simulink model "cartpole"  (R2019b)
settings: Solver=ode15s  StartTime=0.0  StopTime=10  MaxStep=0.01  RelTol=1e-3  EnableMultiTasking=on
values from neighbouring files (symbols this model uses):
  cartpole_init_pose = [-(ground.w/2-1) tire.r+ground.l/2 0]    [cartpole_conf.m]
  g = 9.81    [cartpole_conf.m]
  m_cart = body.m + 2*tire.m + 4*omni.m    [cartpole_conf.m]
  max_steer = 0.42    [cartpole_conf.m]
  max_v = 1    [cartpole_conf.m]
  path = [4.0 0.0 2.0]    [cartpole_conf.m]
  tread = tire.l + body.h    [cartpole_conf.m]
  waypoint_length = 0.05    [cartpole_conf.m]
undefined symbols (not defined in the file or in its folder): body, Body, ground, Ground, LBomni, LCtire, LFomni, omni, RBomni, RCtire, RFomni, sigbuilder_block, stick, Stick, tire, Wall1, Wall2, Wall3, Wall4, X, Y, Z
libraries: sm_lib x106, nesl_utility x18, simulink x5
(part 1 of 4)
settings Model: NumberOfSteps=10  EnablePacing=on  PacingRate=1000  Creator=土屋　一朗  LastModifiedBy=wataru
settings DataIOCC: LimitDataPoints=on  MaxDataPoints=10000
settings OptimizationCC: LifeSpan=inf
settings DebuggingCC: AllowSymbolicDim=off  SFUnexpectedBacktrackingDiag=warning  SFNoUnconditionalDefaultTransitionDiag=warning  SFExecutionAtInitializationDiag=none  ArithmeticOperatorsInVariantConditions=warning
settings SFSimCC: SimUseLocalCustomCode=off  CustomCodeUndefinedFunction=UseInterfaceOnly
settings RTWCC: RTWUseLocalCustomCode=off
settings CodeAppCC: StateflowObjectComments=on
settings GRTTargetCC: TargetLangStandard=C89/C90 (ANSI)  GeneratePreprocessorConditionals=Disable all
settings ConfigComp: CovMetricSettings=dw  CovHtmlReporting=on  CovSaveCumulativeToWorkspaceVar=on  CovSaveSingleToWorkspaceVar=on  CovExternalEMLEnable=off  CovSFcnEnable=off
settings SimscapeCC: SimscapeLogType=all  SimscapeLogSimulationStatistics=on  SimscapeLogDataHistory=10000
settings ExplorerConfigSet: InternalSimMechanicsExplorerSettings="<ExplorerConfiguration><canonicalview>planar_xy</canonicalview><AnimationSetting><BasePlaybackSpeed>1.0</BasePlaybackSpeed><PlaybackSpeedFactor>1.0</PlaybackSpeedFactor></AnimationSetting><TilePanel><TileInfo><Tiles Columns=\"1\" Count=\"1\" Rows=\"1\"><Column Weight=\"1\"/><Row Weight=\"1\"/><Tile Height=\"1\" Width=\"1\" X=\"0\" Y=\"0\"/></Tiles></TileInfo><SceneInfo><SceneViewer><BGColor><R>0.60000002384185791</R><G>0.60000002384185791</G><B>0.60000002384185791</B></BGColor><Camera><DoPerspective>off</DoPerspective><Position><X>5.81087438691202873</X><Y>6.21087454411730366</Y><Z>5.81087458520799416</Z></Position><Center><X>1.96953159822821355e-07</X><Y>0.400000354158434546</Y><Z>3.9524912481825325e-07</Z></Center><Up><X>-0.408248290463863073</X><Y>0.816496580927726145</Y><Z>-0.408248290463863073</Z></Up><ViewLimDist>1</ViewLimDist><YLim>7.91620397355392402</YLim><XLim>7.39244756698608452</XLim></Camera></SceneViewer></SceneInfo></TilePanel><MechEditorPanel><Cameras/><GfxPanelCameraMap/><VideoCreator><PlaybackSpeedRatio>1.0</PlaybackSpeedRatio><FrameRate>30</FrameRate><VideoFormat>Motion JPEG AVI</VideoFormat><FrameSize>auto</FrameSize></VideoCreator></MechEditorPanel></ExplorerConfiguration>"

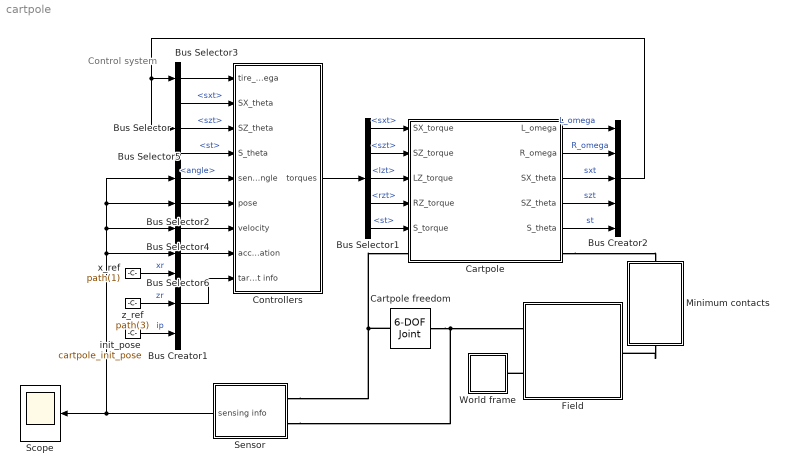
== system cartpole ==
  note: Control system
  Bus Creator1 : BusCreator  Inputs=3
  Bus Creator2 : BusCreator  Inputs=5
  Bus Selector : BusSelector  OutputSignals=sxt,szt,st
  Bus Selector1 : BusSelector  OutputSignals=sxt,szt,lzt,rzt,st
  Bus Selector2 : BusSelector  OutputSignals=x,z  OutputAsBus=on
  Bus Selector3 : BusSelector  OutputSignals=L_omega,R_omega  OutputAsBus=on
  Bus Selector4 : BusSelector  OutputSignals=vx,vz  OutputAsBus=on
  Bus Selector5 : BusSelector  OutputSignals=angle
  Bus Selector6 : BusSelector  OutputSignals=ax,az  OutputAsBus=on
  Cartpole : Subsystem  mask{s_m=stick.m, s_w=stick.w, s_l=stick.l, s_h=stick.h, s_color=stick.color, init_rad=0, b_m=body.m, b_w=body.w, b_l=body.l, b_h=body.h, b_color=body.color, t_m=tire.m, t_r=tire.r, t_l=tire.l, t_color=tire.color, o_m=omni.m, o_r=omni.r, o_color=omni.color}
      mask prompts: s_m "Mass(kg)"; s_w "Width(m)"; s_l "Length(m)"; s_h "Height(m)"; s_color "Color(RGB)"; init_rad "Init rad"; b_m "Mass(kg)"; b_w "Width(m)"; b_l "Length(m)"; b_h "Height(m)"; b_color "Color(RGB)"; t_m "Mass(kg)"; t_r "Radius(m)"; t_l "Length(m)"; t_color "Color(RGB)"; o_m "Mass(kg)"; o_r "Radius(m)"; o_color "Color(RGB)"
      mask DialogControl Container2 Prompt: Stick
      mask DialogControl Container1 Prompt: Body
      mask DialogControl Container3 Prompt: Tire
      mask DialogControl Container11 Prompt: Main
      mask DialogControl Container10 Prompt: omni
      mask Display: image(imread(fullfile('.','images','cartpole.png')));
  Cartpole freedom : sm_lib/Joints/6-DOF Joint  JointMode=Normal  SenseConstraintForce=off  SenseConstraintForceX=off  SenseConstraintForceY=off  SenseConstraintForceZ=off  SenseConstraintTorque=off  SenseConstraintTorqueX=off  SenseConstraintTorqueY=off  SenseConstraintTorqueZ=off  SenseTotalForce=off  SenseTotalForceX=off  SenseTotalForceY=off  SenseTotalForceZ=off  SenseTotalTorque=off  SenseTotalTorqueX=off  SenseTotalTorqueY=off  SenseTotalTorqueZ=off  CompositeWrenchDir=FollowerOnBase  CompositeWrenchFrame=BaseFrame  PxEquilibriumPosition=0  PxEquilibriumPositionUnits=m  PxSpringStiffness=0  PxSpringStiffnessUnits=N/m  PxDampingCoefficient=0  PxDampingCoefficientUnits=N/(m/s)  PxTorqueActuationMode=NoTorque  PxMotionActuationMode=ComputedMotion  PxSensePosition=off  PxSenseVelocity=off  PxSenseAcceleration=off  PxSenseTorqueForce=off  PxSenseLowerLimitTorqueForce=off  PxSenseUpperLimitTorqueForce=off  PxLowerLimitSpecify=off  PxLowerLimitBound=-1  PxLowerLimitBoundUnits=m  PxLowerLimitStiffness=1e6  PxLowerLimitStiffnessUnits=N/m  PxLowerLimitDamping=1e3  PxLowerLimitDampingUnits=N/(m/s)  PxLowerLimitTransitionRegionWidth=1e-4  PxLowerLimitTransitionRegionWidthUnits=m  PxUpperLimitSpecify=off  PxUpperLimitBound=1  PxUpperLimitBoundUnits=m  PxUpperLimitStiffness=1e6  PxUpperLimitStiffnessUnits=N/m  PxUpperLimitDamping=1e3  PxUpperLimitDampingUnits=N/(m/s)  PxUpperLimitTransitionRegionWidth=1e-4  PxUpperLimitTransitionRegionWidthUnits=m  PxPositionTargetSpecify=off  PxPositionTargetPriority=High  PxPositionTargetValue=0  PxPositionTargetValueUnits=m  PxVelocityTargetSpecify=off  PxVelocityTargetPriority=High  PxVelocityTargetValue=0  PxVelocityTargetValueUnits=m/s  PyEquilibriumPosition=0  PyEquilibriumPositionUnits=m  PySpringStiffness=0  PySpringStiffnessUnits=N/m  PyDampingCoefficient=0  PyDampingCoefficientUnits=N/(m/s)  PyTorqueActuationMode=NoTorque  PyMotionActuationMode=ComputedMotion  PySensePosition=off  PySenseVelocity=off  PySenseAcceleration=off  PySenseTorqueForce=off  PySenseLowerLimitTorqueForce=off  PySenseUpperLimitTorqueForce=off  PyLowerLimitSpecify=off  PyLowerLimitBound=-1  PyLowerLimitBoundUnits=m  PyLowerLimitStiffness=1e6  PyLowerLimitStiffnessUnits=N/m  PyLowerLimitDamping=1e3  PyLowerLimitDampingUnits=N/(m/s)  PyLowerLimitTransitionRegionWidth=1e-4  PyLowerLimitTransitionRegionWidthUnits=m  PyUpperLimitSpecify=off  PyUpperLimitBound=1  PyUpperLimitBoundUnits=m  PyUpperLimitStiffness=1e6  PyUpperLimitStiffnessUnits=N/m  PyUpperLimitDamping=1e3  PyUpperLimitDampingUnits=N/(m/s)  PyUpperLimitTransitionRegionWidth=1e-4  PyUpperLimitTransitionRegionWidthUnits=m  PyPositionTargetSpecify=off  PyPositionTargetPriority=High  PyPositionTargetValue=0  PyPositionTargetValueUnits=m  PyVelocityTargetSpecify=off  PyVelocityTargetPriority=High  PyVelocityTargetValue=0  PyVelocityTargetValueUnits=m/s  PzEquilibriumPosition=0  PzEquilibriumPositionUnits=m  PzSpringStiffness=0  PzSpringStiffnessUnits=N/m  PzDampingCoefficient=0  PzDampingCoefficientUnits=N/(m/s)  PzTorqueActuationMode=NoTorque  PzMotionActuationMode=ComputedMotion  PzSensePosition=off  PzSenseVelocity=off  PzSenseAcceleration=off  PzSenseTorqueForce=off  PzSenseLowerLimitTorqueForce=off  PzSenseUpperLimitTorqueForce=off  PzLowerLimitSpecify=off  PzLowerLimitBound=-1  PzLowerLimitBoundUnits=m  PzLowerLimitStiffness=1e6  PzLowerLimitStiffnessUnits=N/m  PzLowerLimitDamping=1e3  PzLowerLimitDampingUnits=N/(m/s)  PzLowerLimitTransitionRegionWidth=1e-4  PzLowerLimitTransitionRegionWidthUnits=m  PzUpperLimitSpecify=off  PzUpperLimitBound=1  PzUpperLimitBoundUnits=m  PzUpperLimitStiffness=1e6  PzUpperLimitStiffnessUnits=N/m  PzUpperLimitDamping=1e3  PzUpperLimitDampingUnits=N/(m/s)  PzUpperLimitTransitionRegionWidth=1e-4  PzUpperLimitTransitionRegionWidthUnits=m  PzPositionTargetSpecify=off  PzPositionTargetPriority=High  PzPositionTargetValue=0  PzPositionTargetValueUnits=m  PzVelocityTargetSpecify=off  PzVelocityTargetPriority=High  PzVelocityTargetValue=0  PzVelocityTargetValueUnits=m/s  SphDefPosRotationMethod=None  SphDefPosRotationAngleUnits=deg  SphDefPosRotationStandardAxis=+Z  SphDefPosRotationAngle=0.0  SphDefPosRotationArbitraryAxis=[0 0 1]  SphDefPosFollAlignAxisA=+X  SphDefPosBaseAlignAxisA=+Y  SphDefPosFollAlignAxisB=+Y  SphDefPosBaseAlignAxisB=+Z  SphDefPosRotationSequenceAxes=FollowerAxes  SphDefPosRotationSequence=XYX  SphDefPosRotationSequenceAngles=[0 0 0]  SphDefPosRotationSequenceAnglesUnits=deg  SphDefPosRotationMatrix=[1 0 0; 0 1 0; 0 0 1]  SphEqPosRotationMethod=None  SphEqPosRotationAngleUnits=deg  SphEqPosRotationStandardAxis=+Z  SphEqPosRotationAngle=0.0  SphEqPosRotationArbitraryAxis=[0 0 1]  SphEqPosFollAlignAxisA=+X  SphEqPosBaseAlignAxisA=+Y  SphEqPosFollAlignAxisB=+Y  SphEqPosBaseAlignAxisB=+Z  SphEqPosRotationSequenceAxes=FollowerAxes  SphEqPosRotationSequence=XYX  SphEqPosRotationSequenceAngles=[0 0 0]  SphEqPosRotationSequenceAnglesUnits=deg  SphEqPosRotationMatrix=[1 0 0; 0 1 0; 0 0 1]  SphSpringStiffness=0  SphSpringStiffnessUnits=N*m/deg  SphDampingCoefficient=0  SphDampingCoefficientUnits=N*m/(deg/s)  SphActuateTorqueX=off  SphActuateTorqueY=off  SphActuateTorqueZ=off  SphActuateTorque=off  SphTorqueActuationMode=NoTorque  SphMotionActuationMode=ComputedMotion  SphActuationFrame=BaseFrame  SphSensePosition=off  SphSenseVelocityX=off  SphSenseVelocityY=off  SphSenseVelocityZ=off  SphSenseVelocity=off  SphSenseAccelerationX=off  SphSenseAccelerationY=off  SphSenseAccelerationZ=off  SphSenseAcceleration=off  SphSenseTorqueX=off  SphSenseTorqueY=off  SphSenseTorqueZ=off  SphSenseTorqueForce=off  SphSenseLowerLimitTorqueMag=off  SphSenseUpperLimitTorqueMag=off  SphSensingFrame=BaseFrame  SphLowerLimitSpecify=off  SphLowerLimitBound=15  SphLowerLimitBoundUnits=deg  SphLowerLimitStiffness=1e4  SphLowerLimitStiffnessUnits=N*m/deg  SphLowerLimitDamping=10  SphLowerLimitDampingUnits=N*m/(deg/s)  SphLowerLimitTransitionRegionWidth=0.1  SphLowerLimitTransitionRegionWidthUnits=deg  SphUpperLimitSpecify=off  SphUpperLimitBound=45  SphUpperLimitBoundUnits=deg  SphUpperLimitStiffness=1e4  SphUpperLimitStiffnessUnits=N*m/deg  SphUpperLimitDamping=10  SphUpperLimitDampingUnits=N*m/(deg/s)  SphUpperLimitTransitionRegionWidth=0.1  SphUpperLimitTransitionRegionWidthUnits=deg  SphPositionTargetRotationMethod=None  SphPositionTargetRotationAngleUnits=deg  SphPositionTargetRotationStandardAxis=+Z  SphPositionTargetRotationAngle=0.0  SphPositionTargetRotationArbitraryAxis=[0 0 1]  SphPositionTargetFollAlignAxisA=+X  SphPositionTargetBaseAlignAxisA=+Y  SphPositionTargetFollAlignAxisB=+Y  SphPositionTargetBaseAlignAxisB=+Z  SphPositionTargetRotationSequenceAxes=FollowerAxes  SphPositionTargetRotationSequence=XYX  SphPositionTargetRotationSequenceAngles=[0 0 0]  SphPositionTargetRotationSequenceAnglesUnits=deg  SphPositionTargetRotationMatrix=[1 0 0; 0 1 0; 0 0 1]  SphPositionTargetSpecify=off  SphPositionTargetPriority=High  SphVelocityTargetValue=[0 0 0]  SphVelocityTargetValueUnits=deg/s  SphVelocityTargetSpecify=off  SphVelocityTargetPriority=High  SphVelocityTargetInFollowerFrame=on
  Controllers : Subsystem
  "Field " : Subsystem  mask{w=ground.w, l=ground.l, h=ground.h, color=ground.color, init=cartpole_init_pose}
      mask prompts: w "Width(m)"; l "Length(m)"; h "Height(m)"; color "Color(RGB)"; init "Cartesian"
      mask DialogControl Container3 Prompt: Ground
      mask DialogControl Container4 Prompt: Init cartpole position
      mask Display: image(imread(fullfile('.','images','field.png')));
  Minimum contacts : Subsystem
  Scope : Scope
  Sensor : Subsystem
  World frame : Subsystem
  init_pose : Constant  Value=cartpole_init_pose  VectorParams1D=off
  x_ref : Constant  Value=path(1)
  z_ref : Constant  Value=path(3)
  wires:
  Controllers/1(torques) -> Bus Selector1/1
  Cartpole/3(SX_theta) -> Bus Creator2/3  "sxt"
  Bus Selector1/1 -> Cartpole/1(SX_torque)  "<sxt>"
  Cartpole/4(SZ_theta) -> Bus Creator2/4  "szt"
  Bus Selector1/2 -> Cartpole/2(SZ_torque)  "<szt>"
  Cartpole/5(S_theta) -> Bus Creator2/5  "st"
  Bus Selector/1 -> Controllers/2(SX_theta)  "<sxt>"
  Bus Selector/2 -> Controllers/3("SZ_theta ")  "<szt>"
  Bus Selector1/3 -> Cartpole/3(LZ_torque)  "<lzt>"
  Bus Selector1/4 -> Cartpole/4(RZ_torque)  "<rzt>"
  Bus Selector1/5 -> Cartpole/5(S_torque)  "<st>"
  Bus Selector/3 -> Controllers/4(S_theta)  "<st>"
  Sensor/1(sensing info) -> Scope/1, Bus Selector5/1, Bus Selector2/1, Bus Selector4/1, Bus Selector6/1
  x_ref/1 -> Bus Creator1/1  "xr"
  z_ref/1 -> Bus Creator1/2  "zr"
  init_pose/1 -> Bus Creator1/3  "ip"
  Bus Creator1/1 -> Controllers/9(target info)
  Bus Selector2/1 -> Controllers/6(pose)
  Bus Selector5/1 -> Controllers/5(sensor_angle)  "<angle>"
  Bus Selector6/1 -> Controllers/8(acceleration)
  Cartpole/1(L_omega) -> Bus Creator2/1  "L_omega"
  Cartpole/2(R_omega) -> Bus Creator2/2  "R_omega"
  Bus Selector4/1 -> Controllers/7(velocity)
  Bus Creator2/1 -> Bus Selector3/1, Bus Selector/1
  Bus Selector3/1 -> Controllers/1(tire_omega)
  connections:
  Cartpole freedom/LConn1 -- Sensor/LConn2 -- "Field "/LConn1
  "Field "/LConn2 -- World frame/LConn1
  Cartpole/RConn1 -- Minimum contacts/RConn1
  Minimum contacts/LConn1 -- "Field "/RConn1
  Cartpole freedom/RConn1 -- Sensor/LConn1 -- Cartpole/LConn1
